simulink model "simulink_discrete_2_R2021a_Ts3"  (R2021a)
settings: Solver=ode23  StartTime=0.0  StopTime=0.7  FixedStep=T1  MaxStep=1E-5  RelTol=1e-3  EnableMultiTasking=on
undefined symbols (not defined in the file): Ts2
libraries: cstblocks x2
settings Model: Creator=Koldo  LastModifiedBy=EIB
settings SolverCC: ShapePreserveControl=EnableAll  ZeroCrossAlgorithm=Adaptive  AlgebraicLoopSolver=TrustRegion  PositivePriorityOrder=on  AutoInsertRateTranBlk=on  InsertRTBMode=Never (minimum delay)
settings DataIOCC: LimitDataPoints=on  SaveFormat=Array  SignalLoggingSaveFormat=ModelDataLogs  ReturnWorkspaceOutputs=off
settings OptimizationCC: ExpressionDepthLimit=2147483647  LifeSpan=inf
settings DebuggingCC: UnderspecifiedInitializationDetection=Classic  MergeDetectMultiDrivingBlocksExec=none  IgnoredZcDiagnostic=none  SolverPrmCheckMsg=warning  FcnCallInpInsideContextMsg=warning  StateNameClashWarn=warning  SFUnexpectedBacktrackingDiag=warning  SFNoUnconditionalDefaultTransitionDiag=warning  SFExecutionAtInitializationDiag=none  SFMachineParentedDataDiag=warning  ArithmeticOperatorsInVariantConditions=warning
settings HardwareCC: ProdBitPerPointer=32  ProdBitPerSizeT=32  ProdBitPerPtrDiffT=32  ProdLargestAtomicFloat=None  ProdIntDivRoundTo=Undefined  ProdEndianess=Unspecified  ProdWordSize=32  ProdHWDeviceType=32-bit Generic
settings ModelReferenceCC: PropagateSignalLabelsOutOfModel=off
settings SFSimCC: SimUseLocalCustomCode=off  CustomCodeUndefinedFunction=UseInterfaceOnly
settings RTWCC: RTWUseLocalCustomCode=off
settings CodeAppCC: StateflowObjectComments=on
settings GRTTargetCC: TargetLangStandard=C89/C90 (ANSI)  CombineOutputUpdateFcns=off  GRTInterface=on
settings ConfigComp: CovMetricSettings=dw  CovSaveCumulativeToWorkspaceVar=on  CovSaveSingleToWorkspaceVar=on  CovExternalEMLEnable=off

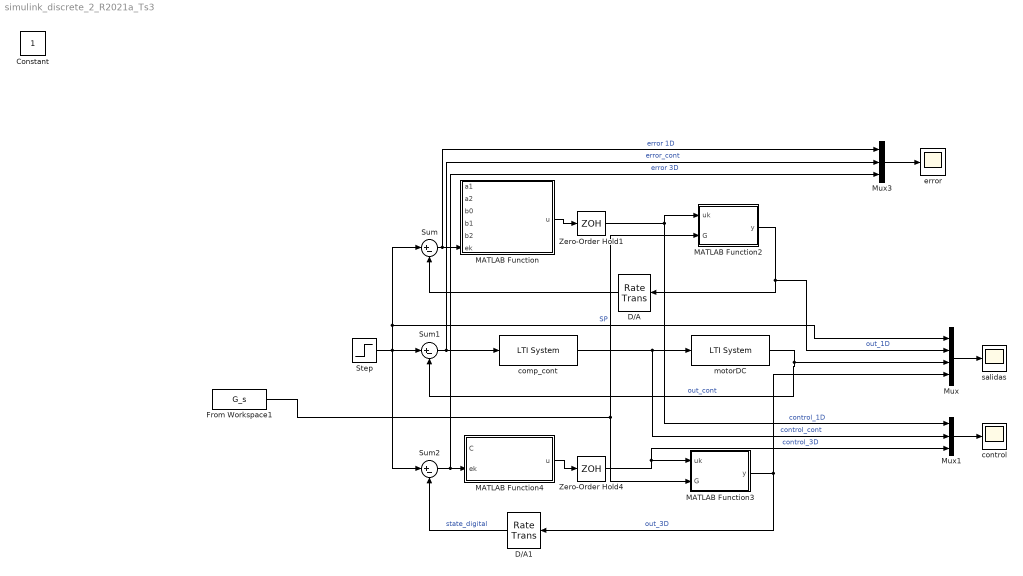
== system simulink_discrete_2_R2021a_Ts3 ==
  D/A : RateTransition  Priority=0  Integrity=off  Deterministic=off  OutPortSampleTime=Ts2
  D/A1 : RateTransition  Integrity=off  Deterministic=off  OutPortSampleTime=Ts2
  From Workspace1 : FromWorkspace  VariableName=G_s  SampleTime=Ts2
  MATLAB Function : MATLAB Function  TreatAsAtomicUnit=on
  MATLAB Function2 : MATLAB Function  TreatAsAtomicUnit=on
  MATLAB Function3 : MATLAB Function  TreatAsAtomicUnit=on
  MATLAB Function4 : MATLAB Function  TreatAsAtomicUnit=on
  Mux : Mux
  Mux1 : Mux  Inputs=3
  Mux3 : Mux  Inputs=3
  Step : Step  Time=0.1  After=pi/2  SampleTime=0
  Sum : Sum  Inputs=|+-
  Sum1 : Sum  Inputs=|+-
  Sum2 : Sum  Inputs=|+-
  Zero-Order Hold1 : ZeroOrderHold  SampleTime=Ts2
  Zero-Order Hold4 : ZeroOrderHold  SampleTime=Ts2
  comp_cont : cstblocks/LTI System  sys=C_s  IC=[]
  control : Scope
  error : Scope
  motorDC : cstblocks/LTI System  sys=G_s  IC=[]
  salidas : Scope
  Constant : Constant  IOType=siggen
  wires:
  Sum/1 -> Mux3/1, MATLAB Function/6(ek)  "error 1D"
  MATLAB Function/1(u) -> Zero-Order Hold1/1
  Sum1/1 -> comp_cont/1, Mux3/2  "error_cont"
  motorDC/1 -> Sum1/2, Mux/3  "out_cont"
  comp_cont/1 -> motorDC/1, Mux1/2  "control_cont"
  Mux/1 -> salidas/1
  Step/1 -> Sum/1, Mux/1, Sum1/1, Sum2/1  "SP"
  Sum2/1 -> MATLAB Function4/2(ek), Mux3/3  "error 3D"
  Zero-Order Hold4/1 -> MATLAB Function3/1(uk), Mux1/3  "control_3D"
  Mux1/1 -> control/1
  MATLAB Function2/1(y) -> D/A/1, Mux/2  "out_1D"
  Zero-Order Hold1/1 -> MATLAB Function2/1(uk), Mux1/1  "control_1D"
  D/A/1 -> Sum/2
  MATLAB Function3/1(y) -> Mux/4, D/A1/1  "out_3D"
  D/A1/1 -> Sum2/2  "state_digital"
  Mux3/1 -> error/1
  MATLAB Function4/1(u) -> Zero-Order Hold4/1
  From Workspace1/1 -> MATLAB Function3/2(G), MATLAB Function2/2(G)

== matlab function simulink_discrete_2_R2021a_Ts3/MATLAB Function ==
  data: a1 input; a2 input; b0 input; b1 input; b2 input; u output; ek input
function u = Cont_dir_1D(a1,a2,b0,b1,b2,ek)

global ek;
%Simula el cálculo de la señal de control del controlador C en tiempo
%discreto. Implementación directa 1D.

%as = C.den{1,1};
%bs = C.num{1,1};

%Parámetros del controlador
%a0 = as(1);
%a1 = as(2);
%a2 = as(3);
%b0 = bs(1);
%b1 = bs(2);
%b2 = bs(3);

%Registros 1D
persistent pk1 pk2

 % Forma canónica (2 registros). Sensible a la cuantificación numérica.
    % uk = b0(ek-a1*pk1-a2*pk2) + b1*pk1 + b2*pk2;
    % Inicializamos los registros (reset)
    if isempty (pk1)
        pk1=0;
    end
    if isempty (pk2)
        pk2=0;
    end
    
    %Realimentación
    ek = setpoints - yk;
    
    %Cálculo de la señal de control
    apk1 = a1*pk1;
    apk2 = a2*pk2;
    pk = ek - apk1 - apk2;
    
    bpk = b0*pk;
    bpk1 = b1*pk1;
    bpk2 = b2*pk2;
    uk = bpk + bpk1 + bpk2;
    
    %Actualizamos los registros
    pk2=pk1;
    pk1=pk;
    u=uk;
y = u;

== matlab function simulink_discrete_2_R2021a_Ts3/MATLAB Function2 ==
  data: uk input; y output; G input
function y = planta(uk, G)

%Simula el comportamiento de la planta G (LTI) en tiempo discreto

as = G.den{1,1};
bs = G.num{1,1};

%Parámetros de la planta
%a0 = as(1);
a1 = as(2);
a2 = as(3);
b0 = bs(1);
b1 = bs(2);
b2 = bs(3);

% y(k)=b0.u(k)+b1*u(k-1)+b2*u(k-2)-a1*y(k-1)-a2*y(k-2);

%Registros
persistent uk1 uk2 yk1 yk2

%Inicializamos los registros
if isempty (yk1)
    yk1=0;
end
if isempty (yk2)
    yk2=0;
end
if isempty (uk1)
    uk1=0;
end
if isempty (uk2)
    uk2=0;
end

%Cálculo de la salida de la planta
% bu0 = b0*uk;
% bu1 = b1*uk1;
% bu2 = b2*uk2;
% ay1 = a1*yk1;
% ay2 = a2*yk2;
% 
% bu01 = bu0+bu1;
% bu012 = bu01+bu2;
% ay12 = ay1+ay2;
% y = bu012 - ay12;

y=b0*uk+b1*uk1+b2*uk2-a1*yk1-a2*yk2;

%Actualizamos los registros
yk2=yk1;
yk1=y;
uk2=uk1;
uk1=uk;

y=y

== matlab function simulink_discrete_2_R2021a_Ts3/MATLAB Function3 ==
  data: uk input; y output; G input
function y = planta(uk, G)

%Simula el comportamiento de la planta G (LTI) en tiempo discreto

as = G.den{1,1};
bs = G.num{1,1};

%Parámetros de la planta
%a0 = as(1);
a1 = as(2);
a2 = as(3);
b0 = bs(1);
b1 = bs(2);
b2 = bs(3);

% y(k)=b0.u(k)+b1*u(k-1)+b2*u(k-2)-a1*y(k-1)-a2*y(k-2);

%Registros
persistent uk1 uk2 yk1 yk2

%Inicializamos los registros
if isempty (yk1)
    yk1=0;
end
if isempty (yk2)
    yk2=0;
end
if isempty (uk1)
    uk1=0;
end
if isempty (uk2)
    uk2=0;
end

%Cálculo de la salida de la planta
% bu0 = b0*uk;
% bu1 = b1*uk1;
% bu2 = b2*uk2;
% ay1 = a1*yk1;
% ay2 = a2*yk2;
% 
% bu01 = bu0+bu1;
% bu012 = bu01+bu2;
% ay12 = ay1+ay2;
% y = bu012 - ay12;

y=b0*uk+b1*uk1+b2*uk2-a1*yk1-a2*yk2;

%Actualizamos los registros
yk2=yk1;
yk1=y;
uk2=uk1;
uk1=uk;

== matlab function simulink_discrete_2_R2021a_Ts3/MATLAB Function4 ==
  data: C input; u output; ek input
function u = Cont_dir_3D(C,ek)
    global ek;
%Simula el cálculo de la señal de control del controlador C en tiempo
%discreto. Implementación directa 1D.

as = C.den{1,1};
bs = C.num{1,1};

%Parámetros del controlador
%a0 = as(1);
a1 = as(2);
a2 = as(3);
b0 = bs(1);
b1 = bs(2);
b2 = bs(3);

%Registros 3D
persistent ek1 ek2 uk1 uk2
% No canónica: cuatro registros
    % u(k) = b0*e(k)+b1*e(k-1)+b2*e(k-2)-a1*u(k-1)-a2*u(k-2)
    
     if isempty (u)
        u=0;
     end 
    if isempty (uk1)
        uk1=0;
     end
     if isempty (uk2)
        uk2=0;
    end
    if isempty (ek1)
        ek1=0;
    end
    if isempty (ek2)
        ek2=0;
    end

    ek= setpoints-u;
    u = b0*ek+b1*ek1+b2*ek2-a1*uk1-a2*uk2;
    uk2=uk1;
    uk1=u;
    ek2=ek1;
    ek1=ek;
y=u
